simulink library "RightIndicator"  (R2015a)
settings: Solver=ode45  StartTime=0.0  StopTime=10.0  RelTol=1e-3
settings Model: Creator=Bruno  LastModifiedBy=Bruno

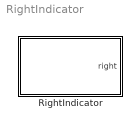
== system RightIndicator ==
  RightIndicator : Stateflow chart  TreatAsAtomicUnit=on

== stateflow chart RightIndicator/RightIndicator ==
  state Off
    entry:
    right=0;
    during: delay(10)
  state On
    entry:
    right=1;
    during: delay(10)
  state delay(time) [function]
    (junction 11) -> (junction 10) [order 1] : [i<time]
    (default) -> (junction 10) : {i=0}
    (junction 10) -> (junction 11) : {i = i + 1}
    (junction 11) -> (junction 12) [order 2]
  On -> Off
  (default) -> Off
  Off -> On
  data: time function_input double size=1; right output double size=1
